simulink library "KERS_SystemModel_lib"  (Simulink 7.7)
settings: Solver=ode45  StartTime=0.0  StopTime=10.0  RelTol=1e-3
undefined symbols (not defined in the file or in its folder): CoeffBrngFric1, CoeffFanDrag1, magnitude
libraries: KERS_SystemModel_lib x4, simulink x1
settings Model: Creator=johannes.krettek  LastModifiedBy=johannes.krettek

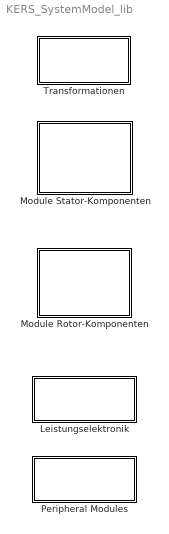
== system KERS_SystemModel_lib ==
  Leistungselektronik : Subsystem
      mask Display: disp('Leistungselektronik')
  Module Rotor-Komponenten : Subsystem
      mask Display: disp('Rotor-Module')
  Module Stator-Komponenten : Subsystem
      mask Display: disp('Stator-Module')
  Peripheral Modules : Subsystem
      mask Display: disp('Peripherie')
  Transformationen : Subsystem
      mask Display: disp('Transformationen')

== system KERS_SystemModel_lib/Leistungselektronik ==
  Dreiecksgenerator : Subsystem
  Dreiphasen-Generator : Subsystem
  Ideale LE : Subsystem
  SKAII2_simple : Subsystem
  Sinus-Dreickes-Modulation : Subsystem  TreatAsAtomicUnit=on

== system KERS_SystemModel_lib/Module Rotor-Komponenten ==
  Lagerreibung Rotor : Subsystem
  Luftreibung Rotor : Subsystem

== system KERS_SystemModel_lib/Module Stator-Komponenten ==
  Drehmomentsberechnung : Subsystem
  Spannungsgleichungen_Stator_einfach : Subsystem
  Spannungsgleichungen_Stator_mit Eisenverlusten : Subsystem  AncestorBlock=KERS_SystemModel_lib/Module Stator-Komponenten/Spannungsgleichungen_Stator_einfach

== system KERS_SystemModel_lib/Peripheral Modules ==
  Position Sensor Model : Subsystem  mask{PosnSens1Offset=0.1, PosnSens2Offset=pi, PosnSensWidth=0.2}
      mask help: Simuliert den idealen Ausgang des Positionssensors, Ausgang=1 wenn die Markeirung detektiert wird, sonst Ausgang=0. Die beiden Markierungen sind "PosnSensWidth" breit und liegen um "PosnSens1Offset" bzw. "PosnSens2Offset" von der Nulllage verschoben. Alle Größen in rad auf dem Gesamtumfang von 2*pi.
  Sensor : Subsystem

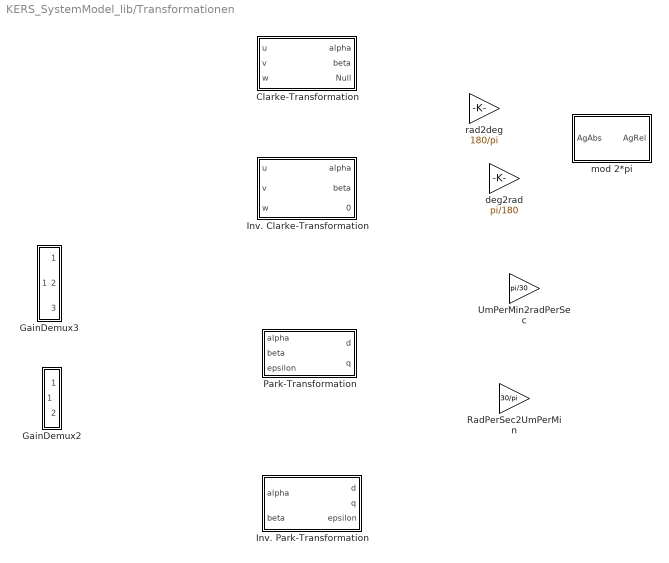
== system KERS_SystemModel_lib/Transformationen ==
  Clarke-Transformation : Subsystem
  GainDemux2 : Subsystem
  GainDemux3 : Subsystem
  Inv. Clarke-Transformation : Subsystem
  Inv. Park-Transformation : Subsystem
  Park-Transformation : Subsystem
  RadPerSec2UmPerMin : Gain  Gain=30/pi
  UmPerMin2radPerSec : Gain  Gain=pi/30
  deg2rad : Gain  Gain=pi/180
  mod 2*pi : Subsystem  mask{tau=2*pi}
      mask Display: fprintf('mod')
  rad2deg : Gain  Gain=180/pi

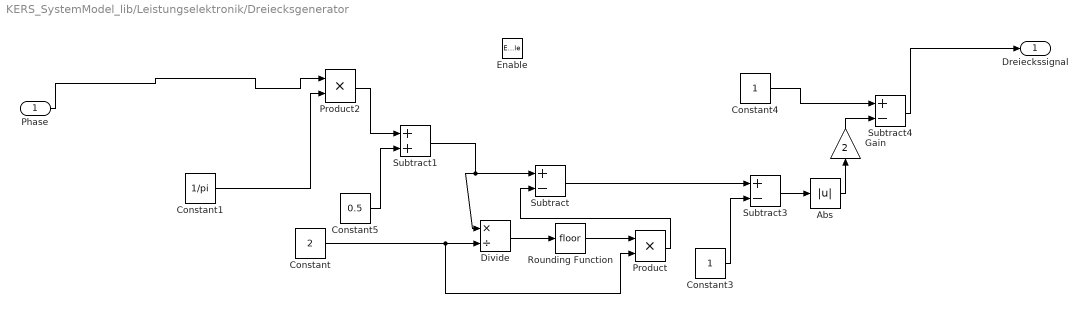
== system KERS_SystemModel_lib/Leistungselektronik/Dreiecksgenerator ==
  Phase : Inport
  Enable : EnablePort  StatesWhenEnabling=reset
  Abs : Abs
  Constant : Constant  Value=2
  Constant1 : Constant  Value=1/pi
  Constant3 : Constant
  Constant4 : Constant
  Constant5 : Constant  Value=0.5
  Divide : Product  Inputs=*/
  Gain : Gain  Gain=2
  Product : Product  RndMeth=Zero
  Product2 : Product  RndMeth=Zero
  Rounding Function : Rounding
  Subtract : Sum  Inputs=+-
  Subtract1 : Sum
  Subtract3 : Sum  Inputs=+-
  Subtract4 : Sum  Inputs=+-
  Dreieckssignal : Outport
  wires:
  Subtract4/1 -> Dreieckssignal/1
  Abs/1 -> Gain/1
  Subtract3/1 -> Abs/1
  Constant4/1 -> Subtract4/1
  Constant3/1 -> Subtract3/2
  Phase/1 -> Product2/1
  Constant/1 -> Divide/2, Product/2
  Divide/1 -> Rounding Function/1
  Subtract/1 -> Subtract3/1
  Rounding Function/1 -> Product/1
  Product/1 -> Subtract/2
  Gain/1 -> Subtract4/2
  Subtract1/1 -> Subtract/1, Divide/1
  Constant5/1 -> Subtract1/2
  Product2/1 -> Subtract1/1
  Constant1/1 -> Product2/2

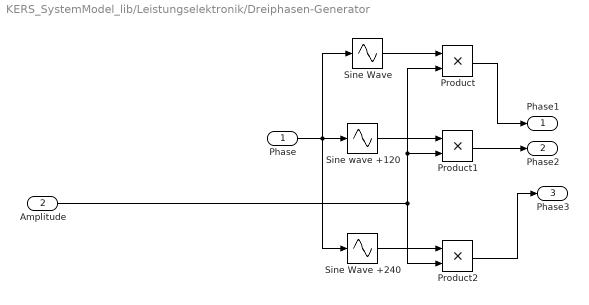
== system KERS_SystemModel_lib/Leistungselektronik/Dreiphasen-Generator ==
  Phase : Inport
  Amplitude : Inport  Port=2
  Product : Product  RndMeth=Zero
  Product1 : Product  RndMeth=Zero
  Product2 : Product  RndMeth=Zero
  Sine Wave : Sin  TimeSource=Use external signal  SampleTime=0
  Sine Wave +240 : Sin  TimeSource=Use external signal  Phase=pi*4/3  SampleTime=0
  Sine wave +120 : Sin  TimeSource=Use external signal  Phase=pi*2/3  SampleTime=0
  Phase1 : Outport
  Phase2 : Outport  Port=2
  Phase3 : Outport  Port=3
  wires:
  Product/1 -> Phase1/1
  Product1/1 -> Phase2/1
  Product2/1 -> Phase3/1
  Amplitude/1 -> Product2/2, Product1/2, Product/2
  Sine Wave/1 -> Product/1
  Sine wave +120/1 -> Product1/1
  Sine Wave +240/1 -> Product2/1
  Phase/1 -> Sine Wave/1, Sine wave +120/1, Sine Wave +240/1

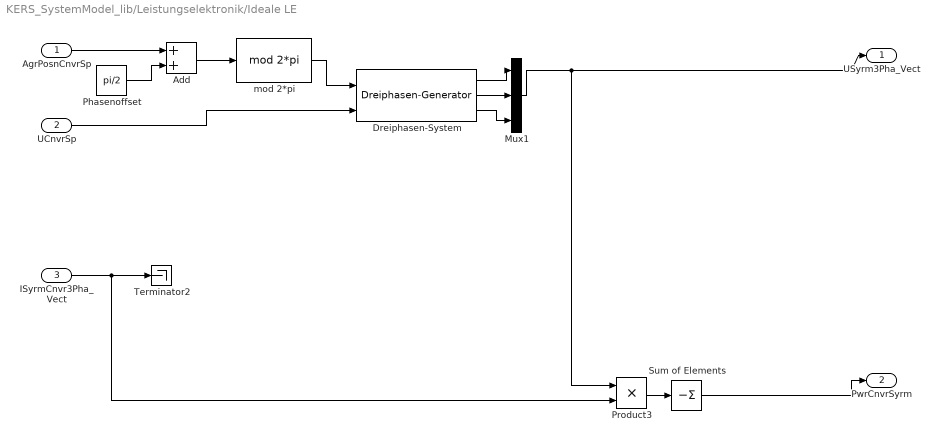
== system KERS_SystemModel_lib/Leistungselektronik/Ideale LE ==
  "AgrPosnCnvrSp " : Inport
  UCnvrSp : Inport  Port=2
  ISyrmCnvr3Pha_Vect : Inport  Port=3
  Add : Sum
  Dreiphasen-System : KERS_SystemModel_lib/Leistungselektronik/Dreiphasen-Generator  SystemSampleTime=-1
  Mux1 : Mux  Inputs=3
  Phasenoffset : Constant  Value=pi/2
  Product3 : Product  RndMeth=Zero
  Sum of Elements : Sum  Inputs=-
  Terminator2 : Terminator
  mod 2*pi : KERS_SystemModel_lib/Transformationen/mod 2*pi  SystemSampleTime=-1
  USyrm3Pha_Vect : Outport
  PwrCnvrSyrm : Outport  Port=2
  wires:
  ISyrmCnvr3Pha_Vect/1 -> Terminator2/1, Product3/2
  Product3/1 -> Sum of Elements/1
  Sum of Elements/1 -> PwrCnvrSyrm/1
  Mux1/1 -> USyrm3Pha_Vect/1, Product3/1
  Add/1 -> mod 2*pi/1
  "AgrPosnCnvrSp "/1 -> Add/1
  Phasenoffset/1 -> Add/2
  mod 2*pi/1 -> Dreiphasen-System/1
  Dreiphasen-System/1 -> Mux1/1
  Dreiphasen-System/2 -> Mux1/2
  Dreiphasen-System/3 -> Mux1/3
  UCnvrSp/1 -> Dreiphasen-System/2

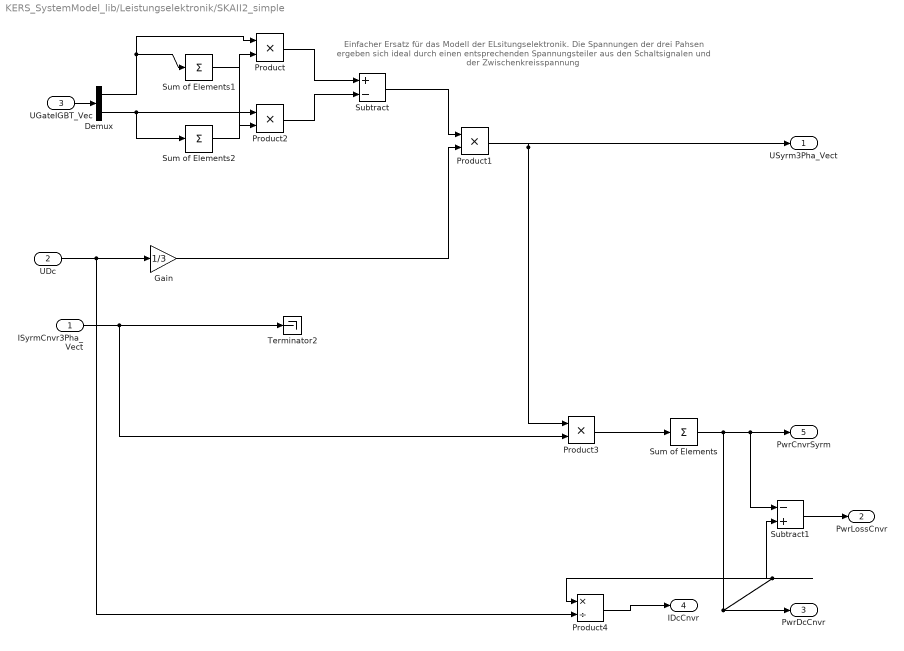
== system KERS_SystemModel_lib/Leistungselektronik/SKAII2_simple ==
  note: Einfacher Ersatz für das Modell der ELsitungselektronik.
      | Die Spannungen der drei Pahsen ergeben sich ideal
      | durch einen entsprechenden Spannungsteiler aus den
      | Schaltsignalen und der Zwischenkreisspannung
  ISyrmCnvr3Pha_Vect : Inport
  UDc : Inport  Port=2
  UGateIGBT_Vec : Inport  Port=3  PortDimensions=6
  Demux : Demux  Outputs=2
  Gain : Gain  Gain=1/3
  Product{,1..3} (4 alike) : Product  RndMeth=Zero
  Product4 : Product  Inputs=*/  RndMeth=Zero
  Subtract : Sum  Inputs=+-
  Subtract1 : Sum  Inputs=-+
  Sum of Elements : Sum  Inputs=+
  Sum of Elements1 : Sum  Inputs=+
  Sum of Elements2 : Sum  Inputs=+
  Terminator2 : Terminator
  USyrm3Pha_Vect : Outport
  PwrLossCnvr : Outport  Port=2
  PwrDcCnvr : Outport  Port=3
  IDcCnvr : Outport  Port=4
  PwrCnvrSyrm : Outport  Port=5
  wires:
  Product4/1 -> IDcCnvr/1
  UDc/1 -> Gain/1, Product4/2
  ISyrmCnvr3Pha_Vect/1 -> Product3/2, Terminator2/1
  Product3/1 -> Sum of Elements/1
  Sum of Elements/1 -> Subtract1/2, Product4/1, PwrDcCnvr/1, Subtract1/1, PwrCnvrSyrm/1
  Product1/1 -> Product3/1, USyrm3Pha_Vect/1
  UGateIGBT_Vec/1 -> Demux/1
  Demux/1 -> Product/1, Sum of Elements1/1
  Demux/2 -> Product2/1, Sum of Elements2/1
  Product/1 -> Subtract/1
  Product2/1 -> Subtract/2
  Gain/1 -> Product1/2
  Subtract/1 -> Product1/1
  Sum of Elements2/1 -> Product/2
  Sum of Elements1/1 -> Product2/2
  Subtract1/1 -> PwrLossCnvr/1

== system KERS_SystemModel_lib/Leistungselektronik/Sinus-Dreickes-Modulation ==
  note: Sinus-Dreick-Modulation (SDM)
      | Durch den Vergleich (<,>) des normierten Sinusverlaufs, dessen Amplitude
      | dem Aussteuergrad der Modulation entspricht, mit einem Dreieckssignal
      | der Amplitude 1 und dreifacher Frequenz, wird ein moduliertes Schaltsignal
      | für den Wechselrichter erzeugt.
  AgrPosnElSp : Inport
  SigSin_Vec : Inport  Port=2
  Detect Decrease : simulink/Logic and Bit Operations/Detect Decrease  SystemSampleTime=-1  vinit=0.0
  Dreiecksgenerator : KERS_SystemModel_lib/Leistungselektronik/Dreiecksgenerator  SystemSampleTime=-1
  Gain : Gain  Gain=-1
  Gain1 : Gain  Gain=3
  Logical Operator : Logic  Operator=NOT  AllPortsSameDT=off  OutDataTypeStr=boolean
  Sign : Signum
  Subtract5 : Sum  Inputs=+-
  SigMod_Vec : Outport
  Dreieckssignal : Outport  Port=2
  wires:
  SigSin_Vec/1 -> Subtract5/1
  Subtract5/1 -> Sign/1
  Sign/1 -> SigMod_Vec/1
  Dreiecksgenerator/1 -> Gain/1
  Gain/1 -> Dreieckssignal/1, Subtract5/2
  Detect Decrease/1 -> Logical Operator/1
  Logical Operator/1 -> Dreiecksgenerator/Enable
  AgrPosnElSp/1 -> Gain1/1, Detect Decrease/1
  Gain1/1 -> Dreiecksgenerator/1

== system KERS_SystemModel_lib/Module Rotor-Komponenten/Lagerreibung Rotor ==
  SpdRtrMec : Inport
  Abs : Abs
  CoeffFricBrng1 Konstante Viskose Lagerreibung : Gain  Gain=CoeffBrngFric1
  TqBrngFric : Outport
  wires:
  SpdRtrMec/1 -> Abs/1
  CoeffFricBrng1 Konstante Viskose Lagerreibung/1 -> TqBrngFric/1
  Abs/1 -> CoeffFricBrng1 Konstante Viskose Lagerreibung/1

== system KERS_SystemModel_lib/Module Rotor-Komponenten/Luftreibung Rotor ==
  SpdRtrMec : Inport
  CoeffFricAir1 Konstante Lüftereffekt : Gain  Gain=CoeffFanDrag1
  Math Function1 : Math  Operator=square  SaturateOnIntegerOverflow=on
  TqFanDrag : Outport
  wires:
  SpdRtrMec/1 -> Math Function1/1
  CoeffFricAir1 Konstante Lüftereffekt/1 -> TqFanDrag/1
  Math Function1/1 -> CoeffFricAir1 Konstante Lüftereffekt/1

== system KERS_SystemModel_lib/Module Stator-Komponenten/Drehmomentsberechnung ==
  note: Berechnung des Drehmoments auf Grundlage der
      | Ströme in DQ-Koordinaten sowie der Polpaarzahl
      | und der Induktivitäten der SyRM.
      | Grundlge für das Moment ist der Reluktanzeffekt.
  ISyrmCnvrDq_d : Inport  PortDimensions=1
  ISyrmCnvrDq_q : Inport  Port=2  PortDimensions=1
  LSyrmCoilDq_d : Inport  Port=3
  LSyrmCoilDq_q : Inport  Port=4
  NrOfPolePairs : Inport  Port=5
  CoeffTqEff : Inport  Port=6
  Gain : Gain  Gain=3/2
  Product : Product  Inputs=5  RndMeth=Zero
  Subtract : Sum  Inputs=+-
  TqFie : Outport
  wires:
  ISyrmCnvrDq_d/1 -> Product/1
  LSyrmCoilDq_d/1 -> Subtract/1
  LSyrmCoilDq_q/1 -> Subtract/2
  Subtract/1 -> Product/3
  Product/1 -> TqFie/1
  Gain/1 -> Product/4
  NrOfPolePairs/1 -> Gain/1
  ISyrmCnvrDq_q/1 -> Product/2
  CoeffTqEff/1 -> Product/5

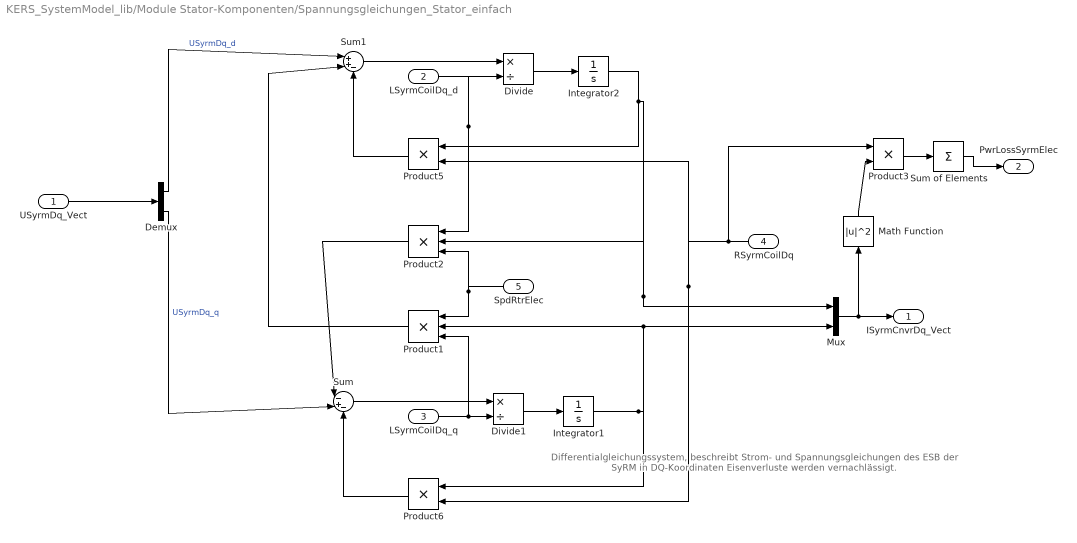
== system KERS_SystemModel_lib/Module Stator-Komponenten/Spannungsgleichungen_Stator_einfach ==
  note: Differentialgleichungssystem, beschreibt Strom- und
      | Spannungsgleichungen des ESB der SyRM in DQ-Koordinaten
      | Eisenverluste werden vernachlässigt.
  USyrmDq_Vect : Inport
  LSyrmCoilDq_d : Inport  Port=2  PortDimensions=1
  LSyrmCoilDq_q : Inport  Port=3  PortDimensions=1
  RSyrmCoilDq : Inport  Port=4  PortDimensions=1
  SpdRtrElec : Inport  Port=5  PortDimensions=1
  Demux : Demux  Outputs=2
  Divide : Product  Inputs=*/
  Divide1 : Product  Inputs=*/
  Integrator1 : Integrator
  Integrator2 : Integrator
  Math Function : Math  Operator=magnitude^2  SaturateOnIntegerOverflow=on
  Mux : Mux  Inputs=2
  Product1 : Product  Inputs=3  RndMeth=Zero  InputSameDT=on
  Product2 : Product  Inputs=3  RndMeth=Zero  InputSameDT=on
  Product3 : Product  RndMeth=Zero
  Product5 : Product  RndMeth=Zero  InputSameDT=on
  Product6 : Product  RndMeth=Zero
  Sum : Sum  Inputs=|-+-
  Sum of Elements : Sum  Inputs=+
  Sum1 : Sum  Inputs=|++-
  ISyrmCnvrDq_Vect : Outport
  PwrLossSyrmElec : Outport  Port=2
  wires:
  Integrator1/1 -> Product6/1, Product1/2, Mux/2
  Divide1/1 -> Integrator1/1
  Demux/1 -> Sum1/1  "USyrmDq_d"
  Integrator2/1 -> Product5/1, Product2/2, Mux/1
  Divide/1 -> Integrator2/1
  Sum1/1 -> Divide/1
  LSyrmCoilDq_d/1 -> Divide/2, Product2/1
  LSyrmCoilDq_q/1 -> Divide1/2, Product1/3
  RSyrmCoilDq/1 -> Product5/2, Product6/2, Product3/1
  Sum/1 -> Divide1/1
  Mux/1 -> ISyrmCnvrDq_Vect/1, Math Function/1
  USyrmDq_Vect/1 -> Demux/1
  SpdRtrElec/1 -> Product2/3, Product1/1
  Product5/1 -> Sum1/3
  Product1/1 -> Sum1/2
  Product6/1 -> Sum/3
  Demux/2 -> Sum/2  "USyrmDq_q"
  Product2/1 -> Sum/1
  Math Function/1 -> Product3/2
  Product3/1 -> Sum of Elements/1
  Sum of Elements/1 -> PwrLossSyrmElec/1

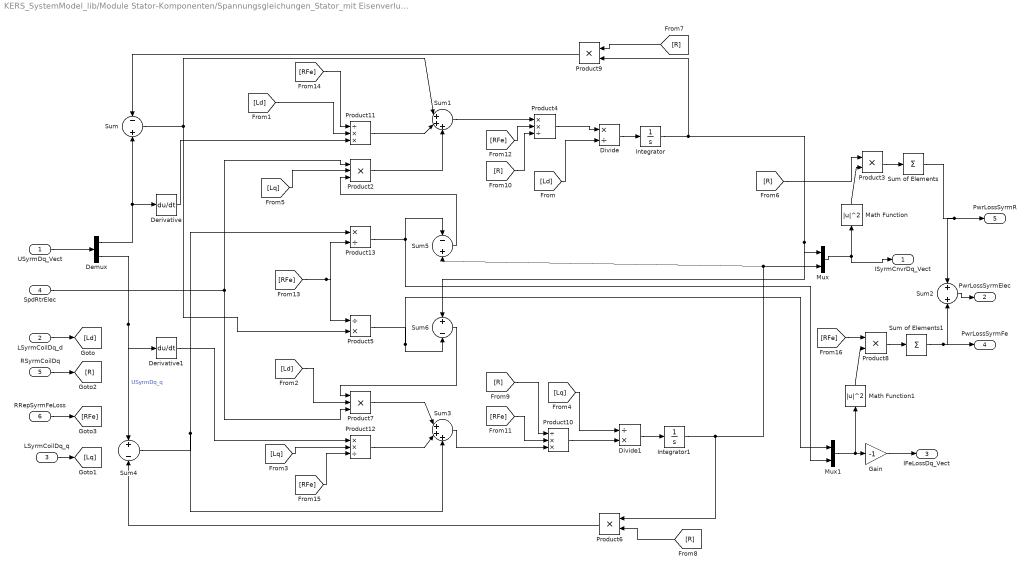
== system KERS_SystemModel_lib/Module Stator-Komponenten/Spannungsgleichungen_Stator_mit Eisenverlusten ==
  USyrmDq_Vect : Inport
  LSyrmCoilDq_d : Inport  Port=2  PortDimensions=1
  LSyrmCoilDq_q : Inport  Port=3  PortDimensions=1
  SpdRtrElec : Inport  Port=4
  RSyrmCoilDq : Inport  Port=5  PortDimensions=1
  RRepSyrmFeLoss : Inport  Port=6  PortDimensions=1
  Demux : Demux  Outputs=2
  Derivative : Derivative
  Derivative1 : Derivative
  Divide : Product  Inputs=*/
  Divide1 : Product  Inputs=/*
  Gain : Gain  Gain=-1
  Integrator : Integrator
  Integrator1 : Integrator
  Math Function : Math  Operator=magnitude^2  SaturateOnIntegerOverflow=on
  Math Function1 : Math  Operator=magnitude^2  SaturateOnIntegerOverflow=on
  Mux : Mux  Inputs=2
  Mux1 : Mux  Inputs=2
  Product10 : Product  Inputs=/**  RndMeth=Zero  InputSameDT=on
  Product11 : Product  Inputs=/**  RndMeth=Zero  InputSameDT=on
  Product12 : Product  Inputs=**/  RndMeth=Zero  InputSameDT=on
  Product13 : Product  Inputs=*/  RndMeth=Zero  InputSameDT=on
  Product2 : Product  Inputs=3  RndMeth=Zero  InputSameDT=on
  Product{3,6,8..9} (4 alike) : Product  RndMeth=Zero
  Product4 : Product  Inputs=**/  RndMeth=Zero  InputSameDT=on
  Product5 : Product  Inputs=/*  RndMeth=Zero  InputSameDT=on
  Product7 : Product  Inputs=3  RndMeth=Zero  InputSameDT=on
  Sum : Sum  Inputs=-+
  Sum of Elements : Sum  Inputs=+
  Sum of Elements1 : Sum  Inputs=+
  Sum1 : Sum  Inputs=|+++
  Sum2 : Sum
  Sum3 : Sum  Inputs=|+++
  Sum4 : Sum  Inputs=+-
  Sum5 : Sum  Inputs=-+
  Sum6 : Sum  Inputs=+-
  ISyrmCnvrDq_Vect : Outport
  PwrLossSyrmElec : Outport  Port=2
  IFeLossDq_Vect : Outport  Port=3
  PwrLossSyrmFe : Outport  Port=4
  PwrLossSyrmR : Outport  Port=5
  wires:
  Product3/1 -> Sum of Elements/1
  Math Function/1 -> Product3/2
  USyrmDq_Vect/1 -> Demux/1
  Mux/1 -> Math Function/1, ISyrmCnvrDq_Vect/1
  Sum of Elements1/1 -> PwrLossSyrmFe/1, Sum2/2
  Product8/1 -> Sum of Elements1/1
  Math Function1/1 -> Product8/2
  Mux1/1 -> Math Function1/1, Gain/1
  Sum of Elements/1 -> PwrLossSyrmR/1, Sum2/1
  Sum2/1 -> PwrLossSyrmElec/1
  Divide/1 -> Integrator/1
  Divide1/1 -> Integrator1/1
  Integrator/1 -> Product9/2, Mux/1, Sum6/1
  Integrator1/1 -> Product6/1, Mux/2, Sum5/2
  Product4/1 -> Divide/1
  Sum1/1 -> Product4/1
  Sum4/1 -> Product13/1, Sum3/3
  Sum/1 -> Sum1/1, Product5/2
  Demux/2 -> Sum4/1, Derivative1/1  "USyrmDq_q"
  Demux/1 -> Sum/2, Derivative/1
  Derivative1/1 -> Product12/1
  Product11/1 -> Sum1/2
  Product12/1 -> Sum3/2
  Product6/1 -> Sum4/2
  Product9/1 -> Sum/1
  SpdRtrElec/1 -> Product7/3, Product2/1
  Product13/1 -> Sum5/1, Mux1/2
  Product5/1 -> Sum6/2, Mux1/1
  Product2/1 -> Sum1/3
  Product7/1 -> Sum3/1
  Gain/1 -> IFeLossDq_Vect/1
  LSyrmCoilDq_d/1 -> [Ld]
  [Ld] -> Divide/2
  [Ld] -> Product7/2
  LSyrmCoilDq_q/1 -> [Lq]
  [Lq] -> Product12/2
  [Lq] -> Divide1/1
  [Lq] -> Product2/2
  RSyrmCoilDq/1 -> [R]
  [R] -> Product3/1
  [R] -> Product9/1
  [R] -> Product6/2
  [R] -> Product10/1
  [R] -> Product4/3
  RRepSyrmFeLoss/1 -> [RFe]
  [RFe] -> Product4/2
  [RFe] -> Product13/2, Product5/1
  [RFe] -> Product12/3
  Product10/1 -> Divide1/2
  Sum3/1 -> Product10/3
  [RFe] -> Product10/2
  [Ld] -> Product11/2
  [RFe] -> Product11/1
  Sum6/1 -> Product7/1
  Sum5/1 -> Product2/3
  [RFe] -> Product8/1
  Derivative/1 -> Product11/3

== system KERS_SystemModel_lib/Peripheral Modules/Position Sensor Model ==
  AgrPosnRtrMec : Inport
  " PosnSens1Offset" : Constant  Value=PosnSens1Offset
  1-D Lookup Table : Lookup_n-D  NumberOfTableDimensions=1  BreakpointsForDimension1="[0 PosnSensWidth  PosnSens2Offset PosnSens2Offset+PosnSensWidth ]"  Table=[1 0 1 0]  InterpMethod=Flat  RndMeth=Simplest  InputSameDT=on
  Sum : Sum  Inputs=|+-
  mod 2*pi : KERS_SystemModel_lib/Transformationen/mod 2*pi  SystemSampleTime=-1  tau=2*pi
  PosnSnsrRaw : Outport
  wires:
  " PosnSens1Offset"/1 -> Sum/2
  AgrPosnRtrMec/1 -> Sum/1
  Sum/1 -> mod 2*pi/1
  mod 2*pi/1 -> 1-D Lookup Table/1
  1-D Lookup Table/1 -> PosnSnsrRaw/1

== system KERS_SystemModel_lib/Peripheral Modules/Sensor ==
  note: Das physikalische Signal wird durch Skalierung, Offset, Begrenzung und Totzeit in eine Messgröße umgesetzt
  Phys. Signal : Inport
  Gain : Gain
  Offset : Constant  Value=0
  Saturation : Saturate  UpperLimit=inf  LowerLimit=-inf
  Sum of Elements : Sum
  Transport Delay : TransportDelay  DelayTime=0
  Signal : Outport
  wires:
  Phys. Signal/1 -> Sum of Elements/1
  Sum of Elements/1 -> Gain/1
  Gain/1 -> Saturation/1
  Offset/1 -> Sum of Elements/2
  Saturation/1 -> Transport Delay/1
  Transport Delay/1 -> Signal/1

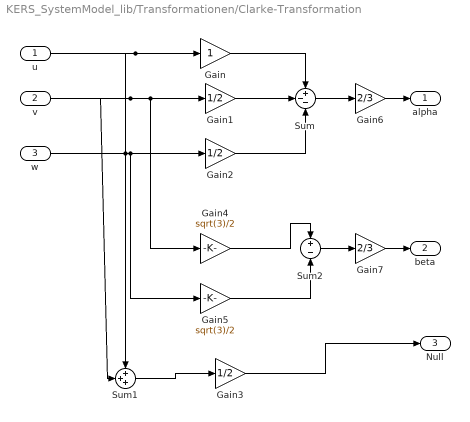
== system KERS_SystemModel_lib/Transformationen/Clarke-Transformation ==
  u : Inport
  v : Inport  Port=2
  w : Inport  Port=3
  Gain : Gain
  Gain1 : Gain  Gain=1/2
  Gain2 : Gain  Gain=1/2
  Gain3 : Gain  Gain=1/2
  Gain4 : Gain  Gain=sqrt(3)/2
  Gain5 : Gain  Gain=sqrt(3)/2
  Gain6 : Gain  Gain=2/3
  Gain7 : Gain  Gain=2/3
  Sum : Sum  Inputs=+--
  Sum1 : Sum  Inputs=+++
  Sum2 : Sum  Inputs=+-
  alpha : Outport
  beta : Outport  Port=2
  Null : Outport  Port=3
  wires:
  Gain/1 -> Sum/1
  Gain1/1 -> Sum/2
  Gain2/1 -> Sum/3
  u/1 -> Gain/1, Sum1/1
  v/1 -> Gain1/1, Gain4/1, Sum1/2
  w/1 -> Gain2/1, Gain5/1, Sum1/3
  Sum/1 -> Gain6/1
  Sum2/1 -> Gain7/1
  Gain6/1 -> alpha/1
  Gain7/1 -> beta/1
  Gain4/1 -> Sum2/1
  Gain5/1 -> Sum2/2
  Gain3/1 -> Null/1
  Sum1/1 -> Gain3/1

== system KERS_SystemModel_lib/Transformationen/GainDemux2 ==
  In1 : Inport
  Demux1 : Demux  Outputs=2
  Gain3 : Gain
  Gain4 : Gain
  Out1 : Outport
  Out2 : Outport  Port=2
  wires:
  Gain4/1 -> Out2/1
  Gain3/1 -> Out1/1
  In1/1 -> Demux1/1
  Demux1/1 -> Gain3/1
  Demux1/2 -> Gain4/1

== system KERS_SystemModel_lib/Transformationen/GainDemux3 ==
  In1 : Inport
  Demux1 : Demux  Outputs=3
  Gain3 : Gain
  Gain4 : Gain
  Gain5 : Gain
  Out1 : Outport
  Out2 : Outport  Port=2
  Out3 : Outport  Port=3
  wires:
  Demux1/1 -> Gain3/1
  Demux1/2 -> Gain4/1
  Demux1/3 -> Gain5/1
  In1/1 -> Demux1/1
  Gain3/1 -> Out1/1
  Gain4/1 -> Out2/1
  Gain5/1 -> Out3/1

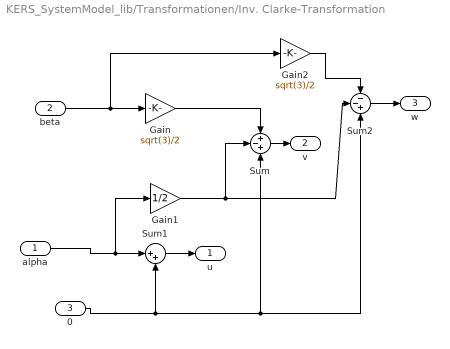
== system KERS_SystemModel_lib/Transformationen/Inv. Clarke-Transformation ==
  alpha : Inport
  beta : Inport  Port=2
  0 : Inport  Port=3
  Gain : Gain  Gain=sqrt(3)/2
  Gain1 : Gain  Gain=1/2
  Gain2 : Gain  Gain=sqrt(3)/2
  Sum : Sum  Inputs=+-+
  Sum1 : Sum  Inputs=|++
  Sum2 : Sum  Inputs=--+
  u : Outport
  v : Outport  Port=2
  w : Outport  Port=3
  wires:
  beta/1 -> Gain/1, Gain2/1
  0/1 -> Sum1/2, Sum/3, Sum2/3
  Sum1/1 -> u/1
  Gain/1 -> Sum/1
  Gain1/1 -> Sum/2, Sum2/2
  Gain2/1 -> Sum2/1
  Sum/1 -> v/1
  Sum2/1 -> w/1
  alpha/1 -> Sum1/1, Gain1/1

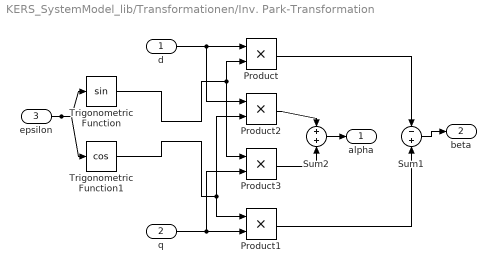
== system KERS_SystemModel_lib/Transformationen/Inv. Park-Transformation ==
  d : Inport
  q : Inport  Port=2
  epsilon : Inport  Port=3
  Product{,1..3} (4 alike) : Product  RndMeth=Zero
  Sum1 : Sum  Inputs=-|+
  Sum2 : Sum  Inputs=+|+
  Trigonometric Function : Trigonometry
  Trigonometric Function1 : Trigonometry  Operator=cos
  alpha : Outport
  beta : Outport  Port=2
  wires:
  Sum2/1 -> alpha/1
  Sum1/1 -> beta/1
  Product3/1 -> Sum2/2
  Product2/1 -> Sum2/1
  Product1/1 -> Sum1/2
  Product/1 -> Sum1/1
  Trigonometric Function1/1 -> Product2/2, Product1/1
  Trigonometric Function/1 -> Product3/1, Product/2
  q/1 -> Product3/2, Product1/2
  d/1 -> Product2/1, Product/1
  epsilon/1 -> Trigonometric Function/1, Trigonometric Function1/1

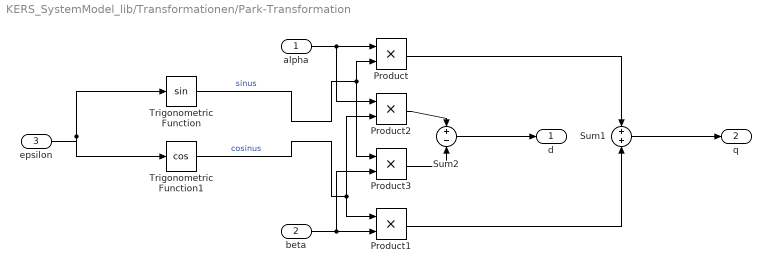
== system KERS_SystemModel_lib/Transformationen/Park-Transformation ==
  alpha : Inport
  beta : Inport  Port=2
  epsilon : Inport  Port=3
  Product{,1..3} (4 alike) : Product  RndMeth=Zero
  Sum1 : Sum  Inputs=+|+
  Sum2 : Sum  Inputs=+|-
  Trigonometric Function : Trigonometry
  Trigonometric Function1 : Trigonometry  Operator=cos
  d : Outport
  q : Outport  Port=2
  wires:
  alpha/1 -> Product/1, Product2/1
  beta/1 -> Product1/2, Product3/2
  Trigonometric Function/1 -> Product/2, Product3/1  "sinus"
  Trigonometric Function1/1 -> Product1/1, Product2/2  "cosinus"
  Product/1 -> Sum1/1
  Product1/1 -> Sum1/2
  Product2/1 -> Sum2/1
  Product3/1 -> Sum2/2
  Sum1/1 -> q/1
  Sum2/1 -> d/1
  epsilon/1 -> Trigonometric Function/1, Trigonometric Function1/1

== system KERS_SystemModel_lib/Transformationen/mod 2*pi ==
  AgAbs : Inport
  Divide : Product  Inputs=*/
  Product : Product  RndMeth=Zero
  Rounding Function : Rounding
  Subtract : Sum  Inputs=+-
  tau : Constant  Value=tau
  AgRel : Outport
  wires:
  Product/1 -> Subtract/2
  Rounding Function/1 -> Product/1
  Subtract/1 -> AgRel/1
  Divide/1 -> Rounding Function/1
  AgAbs/1 -> Subtract/1, Divide/1
  tau/1 -> Product/2, Divide/2
